simulink model "Grua_MC_R2_FFLimitado_06102026"  (R2025b)
settings: Solver=ode23t  StartTime=0.0  StopTime=628  MaxStep=T_s  RelTol=1e-4
InitFcn:
  | addpath(fileparts(get_param(bdroot,'FileName')),'-begin');
  | run(fullfile(fileparts(get_param(bdroot,'FileName')),'definir_buses_variadores.m'));
  | run(fullfile(fileparts(get_param(bdroot,'FileName')),'parametros_ganancias_cascada_29072026.m'));
  | run(fullfile(fileparts(get_param(bdroot,'FileName')),'configurar_modelo_final_hmi.m'));
  | run(fullfile(fileparts(get_param(bdroot,'FileName')),'configurar_parametros_variadores.m'));
  | Pvis.Ts_viz=.04;Pvis.enable=true;Pvis.keepFigureOnTerminate=true;Pvis.hmi.fastDiagnostic=false;
undefined symbols (not defined in the file or in its folder): b_cx, b_cy, b_hb, b_hEb, b_heq, b_t, b_tb, b_teq, b_tw, b_wu, g, H_c, HMI, i_h, i_t, J_heq, J_teq, K_cy, K_tw, k_wu, L_h0, l_hi, M_c_profile, M_s, M_t, MC_FF, nLevels0, omega_hmRATED, r_hd, r_td, slotBlock, T_hbMax, T_hEbMax, T_hmMax, T_s, T_s1, T_tbMax, T_tmMax, tau_hm, tau_tm, traj_duration, traj_x_start, traj_x_target, v_hmaxLoaded, v_hmaxUnloaded, x_tmax, x_tmin, Y_c0, Y_t0, Zbase
libraries: simulink x1, aerolibanimutils x1
(part 2 of 5)

== system Grua_MC_R2_FFLimitado_06102026/Actualizar_Yc ==
  tipo_evento : Inport
  slot_evento : Inport  Port=2
  Trigger : TriggerPort  VariantControl=(inherit)  PortDimensions=1
  Constant : Constant  Value=Zbase
  Constant1 : Constant  Value=slotBlock
  Constant2 : Constant  Value=H_c
  Unit Delay : UnitDelay  InitialCondition=nLevels0  SampleTime=-1  HasFrameUpgradeWarning=on
  update_perfil_std : MATLAB Function  TreatAsAtomicUnit=on
  Y_c : Outport  InitialOutput=Y_c0
  wires:
  update_perfil_std/2(Y_c) -> Y_c/1
  slot_evento/1 -> update_perfil_std/3(slot_evento)
  update_perfil_std/1(nLevels_new) -> Unit Delay/1
  tipo_evento/1 -> update_perfil_std/2(tipo_evento)
  Unit Delay/1 -> update_perfil_std/1(nLevels)
  Constant/1 -> update_perfil_std/4(Zbase)
  Constant1/1 -> update_perfil_std/5(slotBlock)
  Constant2/1 -> update_perfil_std/6(h_std)

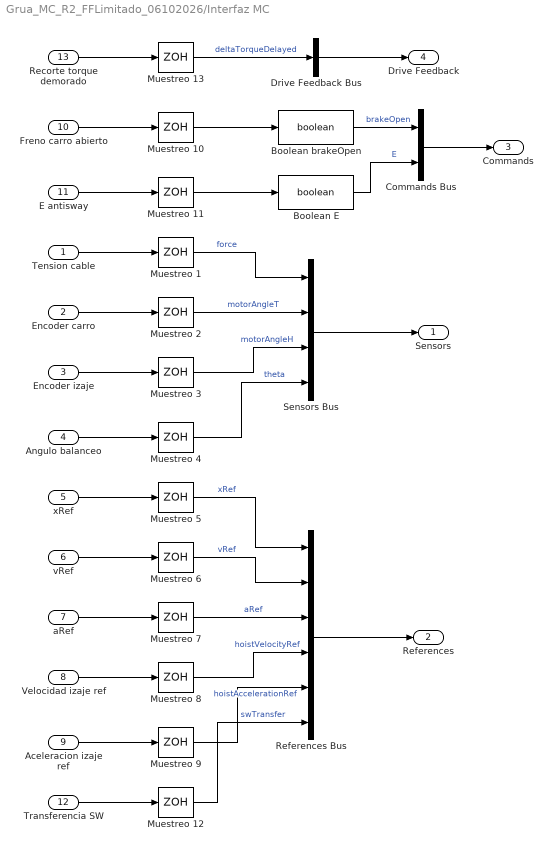
== system Grua_MC_R2_FFLimitado_06102026/Interfaz MC ==
  Tension cable : Inport
  Encoder carro : Inport  Port=2
  Encoder izaje : Inport  Port=3
  Angulo balanceo : Inport  Port=4
  xRef : Inport  Port=5
  vRef : Inport  Port=6
  aRef : Inport  Port=7
  Velocidad izaje ref : Inport  Port=8
  Aceleracion izaje ref : Inport  Port=9
  Freno carro abierto : Inport  Port=10
  E antisway : Inport  Port=11
  Transferencia SW : Inport  Port=12
  Recorte torque demorado : Inport  Port=13
  Boolean E : DataTypeConversion  OutDataTypeStr=boolean  SaturateOnIntegerOverflow=off  RndMeth=Floor
  Boolean brakeOpen : DataTypeConversion  OutDataTypeStr=boolean  SaturateOnIntegerOverflow=off  RndMeth=Floor
  Commands Bus : BusCreator  Inputs=2  OutDataTypeStr=Bus: MCFF_Commands  NonVirtualBus=on
  Drive Feedback Bus : BusCreator  Inputs=1  OutDataTypeStr=Bus: MCFF_DriveFeedback  NonVirtualBus=on
  Muestreo {1..13} (13 alike) : ZeroOrderHold  SampleTime=T_s
  References Bus : BusCreator  Inputs=6  OutDataTypeStr=Bus: MCFF_References  NonVirtualBus=on
  Sensors Bus : BusCreator  Inputs=4  OutDataTypeStr=Bus: MCFF_Sensors  NonVirtualBus=on
  Sensors : Outport
  References : Outport  Port=2
  Commands : Outport  Port=3
  Drive Feedback : Outport  Port=4
  wires:
  Drive Feedback Bus/1 -> Drive Feedback/1
  Muestreo 4/1 -> Sensors Bus/4  "theta"
  E antisway/1 -> Muestreo 11/1
  Recorte torque demorado/1 -> Muestreo 13/1
  Encoder carro/1 -> Muestreo 2/1
  Tension cable/1 -> Muestreo 1/1
  Muestreo 3/1 -> Sensors Bus/3  "motorAngleH"
  Freno carro abierto/1 -> Muestreo 10/1
  xRef/1 -> Muestreo 5/1
  Angulo balanceo/1 -> Muestreo 4/1
  Muestreo 11/1 -> Boolean E/1
  Encoder izaje/1 -> Muestreo 3/1
  Commands Bus/1 -> Commands/1
  vRef/1 -> Muestreo 6/1
  Boolean E/1 -> Commands Bus/2  "E"
  aRef/1 -> Muestreo 7/1
  Velocidad izaje ref/1 -> Muestreo 8/1
  Aceleracion izaje ref/1 -> Muestreo 9/1
  Transferencia SW/1 -> Muestreo 12/1
  Muestreo 13/1 -> Drive Feedback Bus/1  "deltaTorqueDelayed"
  Muestreo 10/1 -> Boolean brakeOpen/1
  Muestreo 1/1 -> Sensors Bus/1  "force"
  Muestreo 2/1 -> Sensors Bus/2  "motorAngleT"
  Muestreo 5/1 -> References Bus/1  "xRef"
  Muestreo 6/1 -> References Bus/2  "vRef"
  Muestreo 7/1 -> References Bus/3  "aRef"
  Muestreo 8/1 -> References Bus/4  "hoistVelocityRef"
  Muestreo 9/1 -> References Bus/5  "hoistAccelerationRef"
  Muestreo 12/1 -> References Bus/6  "swTransfer"
  Boolean brakeOpen/1 -> Commands Bus/1  "brakeOpen"
  Sensors Bus/1 -> Sensors/1
  References Bus/1 -> References/1

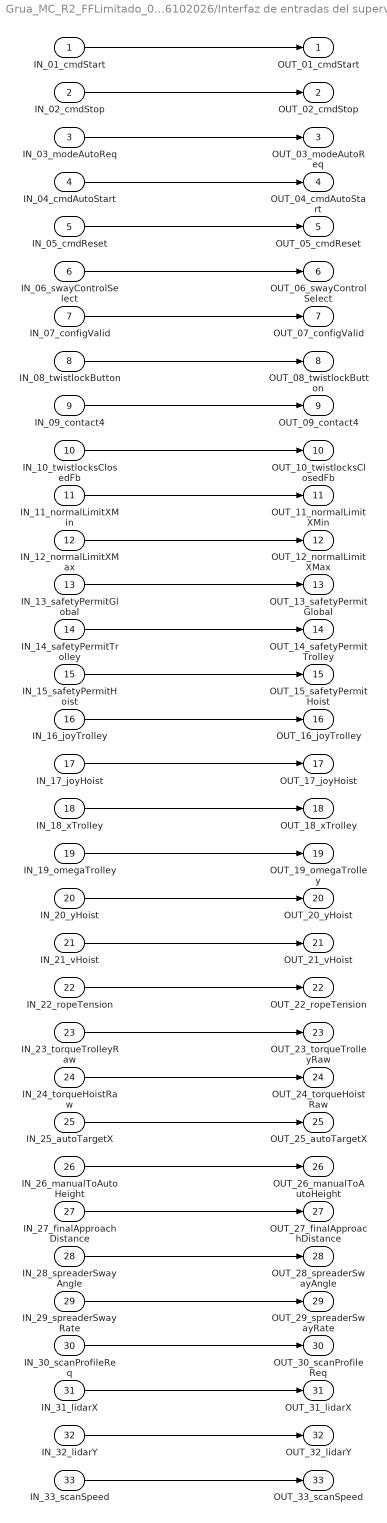
== system Grua_MC_R2_FFLimitado_06102026/Interfaz de entradas del supervisor ==
  IN_01_cmdStart : Inport
  IN_02_cmdStop : Inport  Port=2
  IN_03_modeAutoReq : Inport  Port=3
  IN_04_cmdAutoStart : Inport  Port=4
  IN_05_cmdReset : Inport  Port=5
  IN_06_swayControlSelect : Inport  Port=6
  IN_07_configValid : Inport  Port=7
  IN_08_twistlockButton : Inport  Port=8
  IN_09_contact4 : Inport  Port=9
  IN_10_twistlocksClosedFb : Inport  Port=10
  IN_11_normalLimitXMin : Inport  Port=11
  IN_12_normalLimitXMax : Inport  Port=12
  IN_13_safetyPermitGlobal : Inport  Port=13
  IN_14_safetyPermitTrolley : Inport  Port=14
  IN_15_safetyPermitHoist : Inport  Port=15
  IN_16_joyTrolley : Inport  Port=16
  IN_17_joyHoist : Inport  Port=17
  IN_18_xTrolley : Inport  Port=18
  IN_19_omegaTrolley : Inport  Port=19
  IN_20_yHoist : Inport  Port=20
  IN_21_vHoist : Inport  Port=21
  IN_22_ropeTension : Inport  Port=22
  IN_23_torqueTrolleyRaw : Inport  Port=23
  IN_24_torqueHoistRaw : Inport  Port=24
  IN_25_autoTargetX : Inport  Port=25
  IN_26_manualToAutoHeight : Inport  Port=26
  IN_27_finalApproachDistance : Inport  Port=27
  IN_28_spreaderSwayAngle : Inport  Port=28
  IN_29_spreaderSwayRate : Inport  Port=29
  IN_30_scanProfileReq : Inport  Port=30
  IN_31_lidarX : Inport  Port=31
  IN_32_lidarY : Inport  Port=32
  IN_33_scanSpeed : Inport  Port=33
  OUT_01_cmdStart : Outport
  OUT_02_cmdStop : Outport  Port=2
  OUT_03_modeAutoReq : Outport  Port=3
  OUT_04_cmdAutoStart : Outport  Port=4
  OUT_05_cmdReset : Outport  Port=5
  OUT_06_swayControlSelect : Outport  Port=6
  OUT_07_configValid : Outport  Port=7
  OUT_08_twistlockButton : Outport  Port=8
  OUT_09_contact4 : Outport  Port=9
  OUT_10_twistlocksClosedFb : Outport  Port=10
  OUT_11_normalLimitXMin : Outport  Port=11
  OUT_12_normalLimitXMax : Outport  Port=12
  OUT_13_safetyPermitGlobal : Outport  Port=13
  OUT_14_safetyPermitTrolley : Outport  Port=14
  OUT_15_safetyPermitHoist : Outport  Port=15
  OUT_16_joyTrolley : Outport  Port=16
  OUT_17_joyHoist : Outport  Port=17
  OUT_18_xTrolley : Outport  Port=18
  OUT_19_omegaTrolley : Outport  Port=19
  OUT_20_yHoist : Outport  Port=20
  OUT_21_vHoist : Outport  Port=21
  OUT_22_ropeTension : Outport  Port=22
  OUT_23_torqueTrolleyRaw : Outport  Port=23
  OUT_24_torqueHoistRaw : Outport  Port=24
  OUT_25_autoTargetX : Outport  Port=25
  OUT_26_manualToAutoHeight : Outport  Port=26
  OUT_27_finalApproachDistance : Outport  Port=27
  OUT_28_spreaderSwayAngle : Outport  Port=28
  OUT_29_spreaderSwayRate : Outport  Port=29
  OUT_30_scanProfileReq : Outport  Port=30
  OUT_31_lidarX : Outport  Port=31
  OUT_32_lidarY : Outport  Port=32
  OUT_33_scanSpeed : Outport  Port=33
  wires:
  IN_01_cmdStart/1 -> OUT_01_cmdStart/1
  IN_02_cmdStop/1 -> OUT_02_cmdStop/1
  IN_03_modeAutoReq/1 -> OUT_03_modeAutoReq/1
  IN_04_cmdAutoStart/1 -> OUT_04_cmdAutoStart/1
  IN_05_cmdReset/1 -> OUT_05_cmdReset/1
  IN_06_swayControlSelect/1 -> OUT_06_swayControlSelect/1
  IN_07_configValid/1 -> OUT_07_configValid/1
  IN_08_twistlockButton/1 -> OUT_08_twistlockButton/1
  IN_09_contact4/1 -> OUT_09_contact4/1
  IN_10_twistlocksClosedFb/1 -> OUT_10_twistlocksClosedFb/1
  IN_11_normalLimitXMin/1 -> OUT_11_normalLimitXMin/1
  IN_12_normalLimitXMax/1 -> OUT_12_normalLimitXMax/1
  IN_13_safetyPermitGlobal/1 -> OUT_13_safetyPermitGlobal/1
  IN_14_safetyPermitTrolley/1 -> OUT_14_safetyPermitTrolley/1
  IN_15_safetyPermitHoist/1 -> OUT_15_safetyPermitHoist/1
  IN_16_joyTrolley/1 -> OUT_16_joyTrolley/1
  IN_17_joyHoist/1 -> OUT_17_joyHoist/1
  IN_18_xTrolley/1 -> OUT_18_xTrolley/1
  IN_19_omegaTrolley/1 -> OUT_19_omegaTrolley/1
  IN_20_yHoist/1 -> OUT_20_yHoist/1
  IN_21_vHoist/1 -> OUT_21_vHoist/1
  IN_22_ropeTension/1 -> OUT_22_ropeTension/1
  IN_23_torqueTrolleyRaw/1 -> OUT_23_torqueTrolleyRaw/1
  IN_24_torqueHoistRaw/1 -> OUT_24_torqueHoistRaw/1
  IN_25_autoTargetX/1 -> OUT_25_autoTargetX/1
  IN_26_manualToAutoHeight/1 -> OUT_26_manualToAutoHeight/1
  IN_27_finalApproachDistance/1 -> OUT_27_finalApproachDistance/1
  IN_28_spreaderSwayAngle/1 -> OUT_28_spreaderSwayAngle/1
  IN_29_spreaderSwayRate/1 -> OUT_29_spreaderSwayRate/1
  IN_30_scanProfileReq/1 -> OUT_30_scanProfileReq/1
  IN_31_lidarX/1 -> OUT_31_lidarX/1
  IN_32_lidarY/1 -> OUT_32_lidarY/1
  IN_33_scanSpeed/1 -> OUT_33_scanSpeed/1

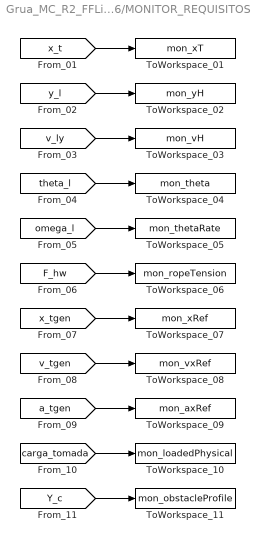
== system Grua_MC_R2_FFLimitado_06102026/MONITOR_REQUISITOS ==
  ToWorkspace_01 : ToWorkspace  VariableName=mon_xT  SaveFormat=Timeseries  SampleTime=-1
      settings: Decimation=10
  ToWorkspace_02 : ToWorkspace  VariableName=mon_yH  SaveFormat=Timeseries  SampleTime=-1
      settings: Decimation=10
  ToWorkspace_03 : ToWorkspace  VariableName=mon_vH  SaveFormat=Timeseries  SampleTime=-1
      settings: Decimation=10
  ToWorkspace_04 : ToWorkspace  VariableName=mon_theta  SaveFormat=Timeseries  SampleTime=-1
      settings: Decimation=10
  ToWorkspace_05 : ToWorkspace  VariableName=mon_thetaRate  SaveFormat=Timeseries  SampleTime=-1
      settings: Decimation=10
  ToWorkspace_06 : ToWorkspace  VariableName=mon_ropeTension  SaveFormat=Timeseries  SampleTime=-1
      settings: Decimation=10
  ToWorkspace_07 : ToWorkspace  VariableName=mon_xRef  SaveFormat=Timeseries  SampleTime=-1
      settings: Decimation=10
  ToWorkspace_08 : ToWorkspace  VariableName=mon_vxRef  SaveFormat=Timeseries  SampleTime=-1
      settings: Decimation=10
  ToWorkspace_09 : ToWorkspace  VariableName=mon_axRef  SaveFormat=Timeseries  SampleTime=-1
      settings: Decimation=10
  ToWorkspace_10 : ToWorkspace  VariableName=mon_loadedPhysical  SaveFormat=Timeseries  SampleTime=-1
      settings: Decimation=10
  ToWorkspace_11 : ToWorkspace  VariableName=mon_obstacleProfile  SaveFormat=Timeseries  SampleTime=-1
      settings: Decimation=10
  wires:
  [x_t] -> ToWorkspace_01/1
  [y_l] -> ToWorkspace_02/1
  [v_ly] -> ToWorkspace_03/1
  [theta_l] -> ToWorkspace_04/1
  [omega_l] -> ToWorkspace_05/1
  [F_hw] -> ToWorkspace_06/1
  [x_tgen] -> ToWorkspace_07/1
  [v_tgen] -> ToWorkspace_08/1
  [a_tgen] -> ToWorkspace_09/1
  [carga_tomada] -> ToWorkspace_10/1
  [Y_c] -> ToWorkspace_11/1

== system Grua_MC_R2_FFLimitado_06102026/Motion Controller ==
  Sensors : Inport  OutDataTypeStr=Bus: MCFF_Sensors
  References : Inport  Port=2  OutDataTypeStr=Bus: MCFF_References
  Commands : Inport  Port=3  OutDataTypeStr=Bus: MCFF_Commands
  Drive Feedback : Inport  Port=4  OutDataTypeStr=Bus: MCFF_DriveFeedback
  Diagnosticos : Subsystem
  Estimadores : MATLAB Function  TreatAsAtomicUnit=on
  MC Carro : MATLAB Function  TreatAsAtomicUnit=on
  MC Izaje : MATLAB Function  TreatAsAtomicUnit=on
  Parameters : Constant  Value=MC_FF  OutDataTypeStr=Bus: MCFF_Parameters  SampleTime=T_s
  T_hm* : Outport
  T_tmcontrolador : Outport  Port=2
  SW aplicada comun : Outport  Port=3
  Estados carro : Outport  Port=4
  Estados izaje : Outport  Port=5
  Diagnosticos carro : Outport  Port=6
  Diagnosticos izaje : Outport  Port=7
  wires:
  MC Carro/1(torque) -> T_tmcontrolador/1
  Sensors/1 -> MC Carro/1(s), MC Izaje/1(s), Estimadores/1(s)
  Parameters/1 -> MC Carro/7(p), MC Izaje/4(p), Estimadores/2(p)
  MC Carro/2(sw) -> SW aplicada comun/1
  Commands/1 -> MC Carro/3(c)
  Drive Feedback/1 -> MC Carro/4(drive)
  Estimadores/1(cart) -> MC Carro/5(est), Estados carro/1
  References/1 -> MC Carro/2(r), MC Izaje/2(r)
  Estimadores/2(hoist) -> MC Izaje/3(est), MC Carro/6(hoist), Estados izaje/1
  MC Carro/3(d) -> Diagnosticos/1(In1), Diagnosticos carro/1
  MC Izaje/1(torque) -> T_hm*/1
  MC Izaje/2(d) -> Diagnosticos izaje/1, Diagnosticos/2(In2)

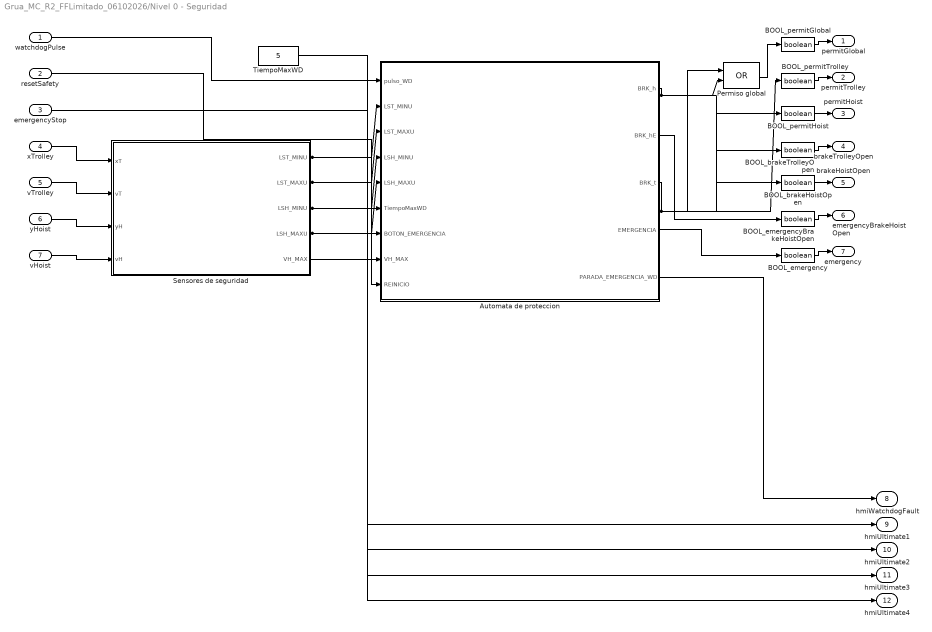
== system Grua_MC_R2_FFLimitado_06102026/Nivel 0 - Seguridad ==
  watchdogPulse : Inport
  resetSafety : Inport  Port=2
  emergencyStop : Inport  Port=3
  xTrolley : Inport  Port=4
  vTrolley : Inport  Port=5
  yHoist : Inport  Port=6
  vHoist : Inport  Port=7
  Automata de proteccion : Stateflow chart  TreatAsAtomicUnit=on
      settings: PortSchema="{\"entries\":[{\"content\":{\"sides\":[{\"content\":{\"connectorIds\":[\"In1\",\"In3\",\"In4\",\"In5\",\"In6\",\"In7\",\"In8\",\"In9\",\"In2\"]},\"type\":\"ConnectorPlacement.EquallySpacedRectSide\",\"uuid\":\"cd0792a4-97ef-4c80-9019-d76753964359\"},{\"content\":{\"connectorIds\":[\"Out1\",\"Out2\",\"Out3\",\"Out4\",\"Out5\"],\"side\":\"RIGHT\"},\"type\":\"ConnectorPlacement.EquallySpacedRectSide\",\"uuid\":\"2986dd5d-2111-4155-8673-f52c044c46ad\"},{\"content\":{\"side\":\"TOP\"},\"type\":\"ConnectorPlacement.EquallySpacedRectSide\",\"uuid\":\"d52e82c5-c118-49d3-899a-ea936e299c34\"}]},\"type\":\"ConnectorPlacement.EquallySpacedConnector\",\"uuid\":\"580a1a82-6a30-4652-9187-78ca47e5d1d9\"}],\"packageUris\":[\"http://schema.mathworks.com/mf0/Connector/R2020b\"],\"version\":\"1.0\"}"
  BOOL_brakeHoistOpen : DataTypeConversion  OutDataTypeStr=boolean  SaturateOnIntegerOverflow=off  RndMeth=Floor
  BOOL_brakeTrolleyOpen : DataTypeConversion  OutDataTypeStr=boolean  SaturateOnIntegerOverflow=off  RndMeth=Floor
  BOOL_emergency : DataTypeConversion  OutDataTypeStr=boolean  SaturateOnIntegerOverflow=off  RndMeth=Floor
  BOOL_emergencyBrakeHoistOpen : DataTypeConversion  OutDataTypeStr=boolean  SaturateOnIntegerOverflow=off  RndMeth=Floor
  BOOL_permitGlobal : DataTypeConversion  OutDataTypeStr=boolean  SaturateOnIntegerOverflow=off  RndMeth=Floor
  BOOL_permitHoist : DataTypeConversion  OutDataTypeStr=boolean  SaturateOnIntegerOverflow=off  RndMeth=Floor
  BOOL_permitTrolley : DataTypeConversion  OutDataTypeStr=boolean  SaturateOnIntegerOverflow=off  RndMeth=Floor
  Permiso global : Logic  Operator=OR  AllPortsSameDT=off  OutDataTypeStr=boolean
  Sensores de seguridad : MATLAB Function  TreatAsAtomicUnit=on
  TiempoMaxWD : Constant  Value=5  OutDataTypeStr=double
  permitGlobal : Outport
  permitTrolley : Outport  Port=2
  permitHoist : Outport  Port=3
  brakeTrolleyOpen : Outport  Port=4
  brakeHoistOpen : Outport  Port=5
  emergencyBrakeHoistOpen : Outport  Port=6
  emergency : Outport  Port=7
  hmiWatchdogFault : Outport  Port=8
  hmiUltimate1 : Outport  Port=9
  hmiUltimate2 : Outport  Port=10
  hmiUltimate3 : Outport  Port=11
  hmiUltimate4 : Outport  Port=12
  wires:
  xTrolley/1 -> Sensores de seguridad/1(xT)
  vTrolley/1 -> Sensores de seguridad/2(vT)
  yHoist/1 -> Sensores de seguridad/3(yH)
  vHoist/1 -> Sensores de seguridad/4(vH)
  watchdogPulse/1 -> Automata de proteccion/1(pulso_WD)
  resetSafety/1 -> Automata de proteccion/2(REINICIO)
  Sensores de seguridad/1(LST_MINU) -> Automata de proteccion/3(LST_MINU), hmiUltimate1/1
  Sensores de seguridad/2(LST_MAXU) -> Automata de proteccion/4(LST_MAXU), hmiUltimate2/1
  Sensores de seguridad/3(LSH_MINU) -> Automata de proteccion/5(LSH_MINU), hmiUltimate3/1
  Sensores de seguridad/4(LSH_MAXU) -> Automata de proteccion/6(LSH_MAXU), hmiUltimate4/1
  TiempoMaxWD/1 -> Automata de proteccion/7(TiempoMaxWD)
  emergencyStop/1 -> Automata de proteccion/8(BOTON_EMERGENCIA)
  Sensores de seguridad/5(VH_MAX) -> Automata de proteccion/9(VH_MAX)
  Automata de proteccion/3(BRK_t) -> Permiso global/1, BOOL_permitTrolley/1, BOOL_brakeTrolleyOpen/1
  Automata de proteccion/1(BRK_h) -> Permiso global/2, BOOL_permitHoist/1, BOOL_brakeHoistOpen/1
  Permiso global/1 -> BOOL_permitGlobal/1
  BOOL_permitGlobal/1 -> permitGlobal/1
  BOOL_permitTrolley/1 -> permitTrolley/1
  BOOL_permitHoist/1 -> permitHoist/1
  BOOL_brakeTrolleyOpen/1 -> brakeTrolleyOpen/1
  BOOL_brakeHoistOpen/1 -> brakeHoistOpen/1
  Automata de proteccion/2(BRK_hE) -> BOOL_emergencyBrakeHoistOpen/1
  BOOL_emergencyBrakeHoistOpen/1 -> emergencyBrakeHoistOpen/1
  Automata de proteccion/4(EMERGENCIA) -> BOOL_emergency/1
  BOOL_emergency/1 -> emergency/1
  Automata de proteccion/5(PARADA_EMERGENCIA_WD) -> hmiWatchdogFault/1

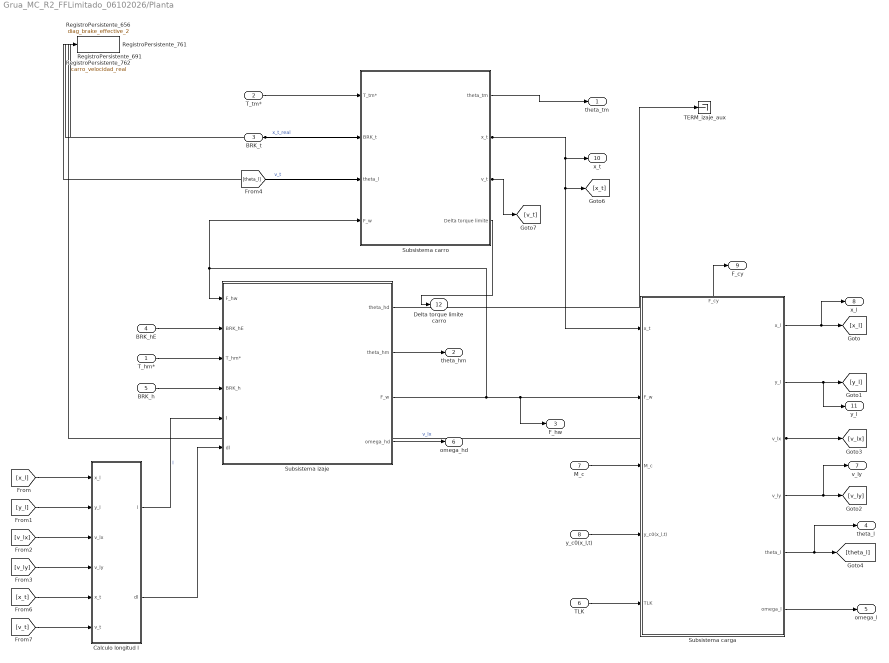
== system Grua_MC_R2_FFLimitado_06102026/Planta ==
  T_hm* : Inport
  T_tm* : Inport  Port=2
  BRK_t : Inport  Port=3
  BRK_hE : Inport  Port=4
  BRK_h : Inport  Port=5
  TLK : Inport  Port=6
  M_c : Inport  Port=7
  y_c0(x_l,t) : Inport  Port=8
  Calculo longitud l : Subsystem
  RegistroPersistente_656 : ToWorkspace  VariableName=diag_brake_effective_2  SaveFormat=Timeseries  SampleTime=-1
      settings: Decimation=10
  RegistroPersistente_691 : ToWorkspace  VariableName=v_lx  SaveFormat=Timeseries  SampleTime=-1
      settings: Decimation=10
  RegistroPersistente_761 : ToWorkspace  VariableName=x_t_real  SaveFormat=Timeseries  SampleTime=-1
      settings: Decimation=10
  RegistroPersistente_762 : ToWorkspace  VariableName=carro_velocidad_real  SaveFormat=Timeseries  SampleTime=-1
      settings: Decimation=10
  Subsistema carga : Subsystem
      settings: PortSchema="{\"entries\":[{\"content\":{\"sides\":[{\"content\":{\"connectorIds\":[\"In1\",\"In2\",\"In3\",\"In4\",\"In5\"]},\"type\":\"ConnectorPlacement.EquallySpacedRectSide\",\"uuid\":\"47edabbd-243a-4b83-941f-e4392c1d00a7\"},{\"content\":{\"connectorIds\":[\"Out1\",\"Out2\",\"Out3\",\"Out4\",\"Out5\",\"Out6\"],\"side\":\"RIGHT\"},\"type\":\"ConnectorPlacement.EquallySpacedRectSide\",\"uuid\":\"f3c5bb4b-ba1f-46ef-b9da-f46dde7ba679\"},{\"content\":{\"connectorIds\":[\"Out7\"],\"side\":\"TOP\"},\"type\":\"ConnectorPlacement.EquallySpacedRectSide\",\"uuid\":\"99c64c8e-1061-494c-a8fc-4982bc564791\"}]},\"type\":\"ConnectorPlacement.EquallySpacedConnector\",\"uuid\":\"f8d59f7d-b4a0-41b3-9b68-cb1adbf574c0\"}],\"packageUris\":[\"http://schema.mathworks.com/mf0/Connector/R2020b\"],\"version\":\"1.0\"}"
  Subsistema carro : Subsystem
  Subsistema izaje : Subsystem
  TERM_izaje_aux : Terminator
  theta_tm : Outport
  theta_hm : Outport  Port=2
  F_hw : Outport  Port=3
  theta_l : Outport  Port=4
  omega_l : Outport  Port=5
  omega_hd : Outport  Port=6
  v_ly : Outport  Port=7
  x_l : Outport  Port=8
  F_cy : Outport  Port=9
  x_t : Outport  Port=10
  y_l : Outport  Port=11
  Delta torque limite carro : Outport  Port=12
  wires:
  y_c0(x_l,t)/1 -> Subsistema carga/4(y_c0(x_l,t))
  [x_t] -> Calculo longitud l/5(x_t)
  Subsistema izaje/3(F_w) -> Subsistema carro/4(F_w), Subsistema izaje/1(F_hw), F_hw/1, Subsistema carga/2(F_w)
  Subsistema carro/2(x_t) -> x_t/1, Subsistema carga/1(x_t), [x_t], RegistroPersistente_761/1  "x_t_real"
  [y_l] -> Calculo longitud l/2(y_l)
  BRK_hE/1 -> Subsistema izaje/2(BRK_hE)
  T_hm*/1 -> Subsistema izaje/3(T_hm*)
  T_tm*/1 -> Subsistema carro/1(T_tm*)
  Subsistema carga/3(v_lx) -> [v_lx], RegistroPersistente_691/1  "v_lx"
  [v_ly] -> Calculo longitud l/4(v_ly)
  Subsistema carga/2(y_l) -> [y_l], y_l/1
  Subsistema carga/4(v_ly) -> v_ly/1, [v_ly]
  Subsistema carga/1(x_l) -> x_l/1, [x_l]
  Subsistema carga/6(omega_l) -> omega_l/1
  [theta_l] -> Subsistema carro/3(theta_l)
  Calculo longitud l/2(dl) -> Subsistema izaje/6(dl)
  [v_lx] -> Calculo longitud l/3(v_lx)
  BRK_t/1 -> Subsistema carro/2(BRK_t), RegistroPersistente_656/1
  M_c/1 -> Subsistema carga/3(M_c)
  [x_l] -> Calculo longitud l/1(x_l)
  Subsistema carro/3(v_t) -> [v_t], RegistroPersistente_762/1  "v_t"
  Calculo longitud l/1(l) -> Subsistema izaje/5(l)  "l"
  [v_t] -> Calculo longitud l/6(v_t)
  BRK_h/1 -> Subsistema izaje/4(BRK_h)
  Subsistema izaje/4(omega_hd) -> omega_hd/1
  Subsistema carro/1(theta_tm) -> theta_tm/1
  Subsistema izaje/2(theta_hm) -> theta_hm/1
  Subsistema carga/5(theta_l) -> theta_l/1, [theta_l]
  Subsistema carga/7(F_cy) -> F_cy/1
  TLK/1 -> Subsistema carga/5(TLK)
  Subsistema izaje/1(theta_hd) -> TERM_izaje_aux/1
  Subsistema carro/4(Delta torque limite) -> Delta torque limite carro/1

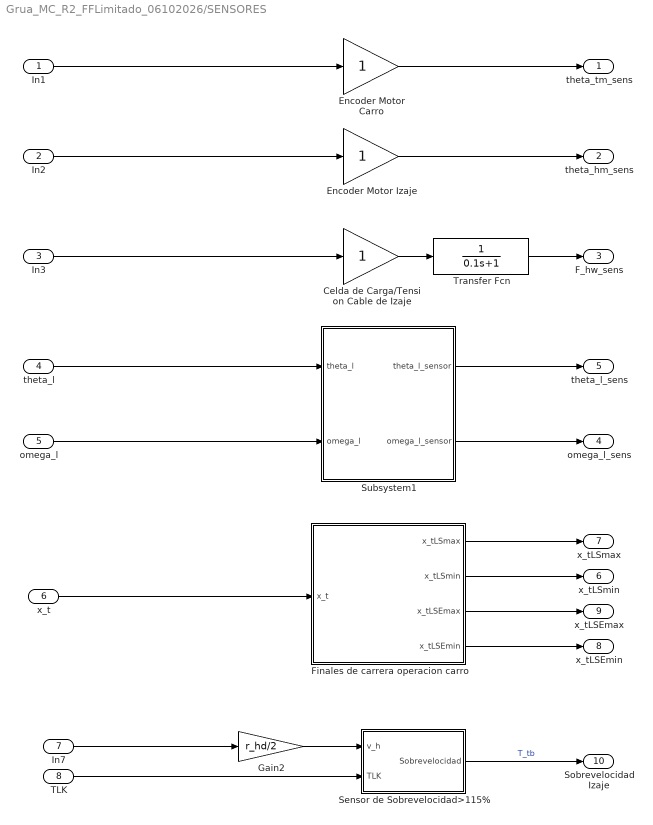
== system Grua_MC_R2_FFLimitado_06102026/SENSORES ==
  In1 : Inport
  In2 : Inport  Port=2
  In3 : Inport  Port=3
  theta_l : Inport  Port=4
  omega_l : Inport  Port=5
  x_t : Inport  Port=6
  In7 : Inport  Port=7
  TLK : Inport  Port=8
  Celda de Carga/Tension Cable de Izaje : Gain
  Encoder Motor Carro : Gain
  Encoder Motor Izaje : Gain
  Finales de carrera operacion carro : Subsystem
  Gain2 : Gain  Gain=r_hd/2
  Sensor de Sobrevelocidad>115% : Subsystem
  Subsystem1 : Subsystem
  Transfer Fcn : TransferFcn  Denominator=[0.1 1]
  theta_tm_sens : Outport
  theta_hm_sens : Outport  Port=2
  F_hw_sens : Outport  Port=3
  omega_l_sens : Outport  Port=4
  theta_l_sens : Outport  Port=5
  x_tLSmin : Outport  Port=6
  x_tLSmax : Outport  Port=7
  x_tLSEmin : Outport  Port=8
  x_tLSEmax : Outport  Port=9
  Sobrevelocidad Izaje : Outport  Port=10
  wires:
  In1/1 -> Encoder Motor Carro/1
  Finales de carrera operacion carro/2(x_tLSmin) -> x_tLSmin/1
  Finales de carrera operacion carro/4(x_tLSEmin) -> x_tLSEmin/1
  Finales de carrera operacion carro/3(x_tLSEmax) -> x_tLSEmax/1
  Celda de Carga/Tension Cable de Izaje/1 -> Transfer Fcn/1
  Subsystem1/2(omega_l_sensor) -> omega_l_sens/1
  Encoder Motor Carro/1 -> theta_tm_sens/1
  Subsystem1/1(theta_l_sensor) -> theta_l_sens/1
  Sensor de Sobrevelocidad>115%/1(Sobrevelocidad) -> Sobrevelocidad Izaje/1  "T_tb"
  Gain2/1 -> Sensor de Sobrevelocidad>115%/1(v_h)
  x_t/1 -> Finales de carrera operacion carro/1(x_t)
  Encoder Motor Izaje/1 -> theta_hm_sens/1
  Finales de carrera operacion carro/1(x_tLSmax) -> x_tLSmax/1
  TLK/1 -> Sensor de Sobrevelocidad>115%/2(TLK)
  theta_l/1 -> Subsystem1/1(theta_l)
  In3/1 -> Celda de Carga/Tension Cable de Izaje/1
  omega_l/1 -> Subsystem1/2(omega_l)
  In2/1 -> Encoder Motor Izaje/1
  In7/1 -> Gain2/1
  Transfer Fcn/1 -> F_hw_sens/1

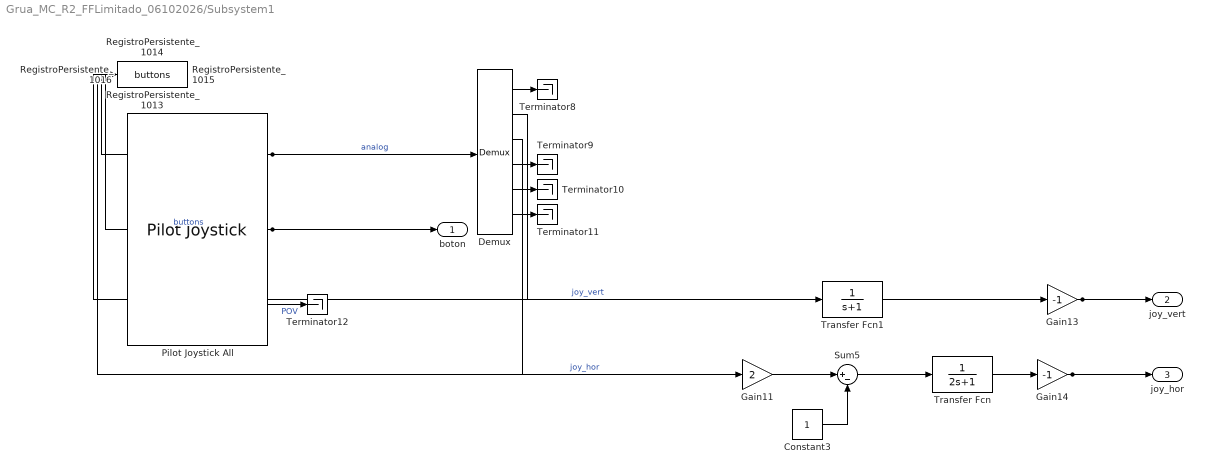
== system Grua_MC_R2_FFLimitado_06102026/Subsystem1 ==
  Constant3 : Constant
  Demux : Demux  Outputs=6
  Gain11 : Gain  Gain=2
  Gain13 : Gain  Gain=-1
  Gain14 : Gain  Gain=-1
  Pilot Joystick All : aerolibanimutils/Pilot Joystick  JoystickID=None  OutputConfiguration=AllOutputs  SampleTime=1/3000
      settings: LibrarySourceBlock=aerolibanimutils/Pilot Joystick All
  RegistroPersistente_1013 : ToWorkspace  VariableName=joy_vert  SaveFormat=Timeseries  SampleTime=-1
      settings: Decimation=10
  RegistroPersistente_1014 : ToWorkspace  VariableName=joy_hor  SaveFormat=Timeseries  SampleTime=-1
      settings: Decimation=10
  RegistroPersistente_1015 : ToWorkspace  VariableName=analog  SaveFormat=Timeseries  SampleTime=-1
      settings: Decimation=10
  RegistroPersistente_1016 : ToWorkspace  VariableName=buttons  SaveFormat=Timeseries  SampleTime=-1
      settings: Decimation=10
  Sum5 : Sum  Inputs=|+-
  Terminator{8..12} (5 alike) : Terminator
  Transfer Fcn : TransferFcn  Denominator=[2 1]
  Transfer Fcn1 : TransferFcn  Denominator=[1 1]
  boton : Outport
  joy_vert : Outport  Port=2
  joy_hor : Outport  Port=3
  wires:
  Demux/5 -> Terminator10/1
  Pilot Joystick All/2 -> boton/1, RegistroPersistente_1016/1  "buttons"
  Demux/2 -> Transfer Fcn1/1
  Constant3/1 -> Sum5/2
  Pilot Joystick All/3 -> Terminator12/1  "POV"
  Transfer Fcn/1 -> Gain14/1
  Demux/1 -> Terminator8/1
  Sum5/1 -> Transfer Fcn/1
  Gain11/1 -> Sum5/1
  Demux/3 -> Gain11/1
  Transfer Fcn1/1 -> Gain13/1
  Pilot Joystick All/1 -> Demux/1, RegistroPersistente_1015/1  "analog"
  Demux/4 -> Terminator9/1
  Demux/6 -> Terminator11/1
  Gain14/1 -> joy_hor/1, RegistroPersistente_1014/1  "joy_hor"
  Gain13/1 -> joy_vert/1, RegistroPersistente_1013/1  "joy_vert"

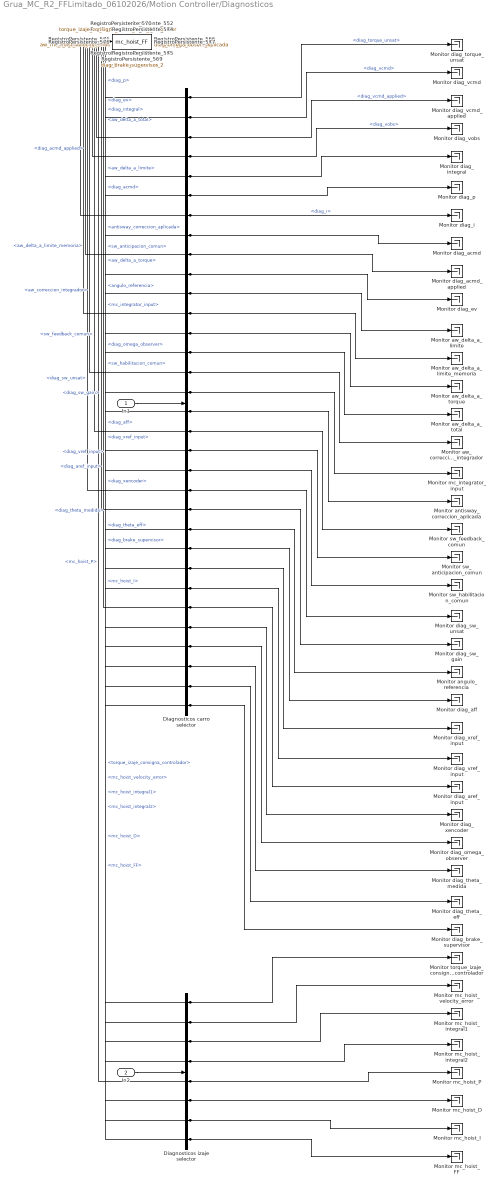
== system Grua_MC_R2_FFLimitado_06102026/Motion Controller/Diagnosticos ==
  In1 : Inport
  In2 : Inport  Port=2
  Diagnosticos carro selector : BusSelector  OutputSignals=diag_torque_unsat,diag_vcmd,diag_vcmd_applied,diag_vobs,diag_integral,diag_p,diag_i,diag_acmd,diag_acmd_applied,diag_ev,aw_delta_a_limite,aw_delta_a_limite_memoria,aw_delta_a_torque,aw_delta_a_total,aw_correccion_integrador,mc_integrator_input,antisway_correccion_aplicada,sw_feedback_comun,sw_anticipacion_comun,sw_habilitacion_comun,diag_sw_unsat,diag_sw_gain,angulo_referencia,diag_aff,diag_xref_input,diag_vref_input,diag_aref_input,diag_xencoder,diag_omega_observer,diag_theta_medida,diag_theta_eff,diag_brake_supervisor
  Diagnosticos izaje selector : BusSelector  OutputSignals=torque_izaje_consigna_controlador,mc_hoist_velocity_error,mc_hoist_integral1,mc_hoist_integral2,mc_hoist_P,mc_hoist_D,mc_hoist_I,mc_hoist_FF
  Monitor angulo_referencia : Terminator
  Monitor antisway_correccion_aplicada : Terminator
  Monitor aw_correccion_integrador : Terminator
  Monitor aw_delta_a_limite : Terminator
  Monitor aw_delta_a_limite_memoria : Terminator
  Monitor aw_delta_a_torque : Terminator
  Monitor aw_delta_a_total : Terminator
  Monitor diag_acmd : Terminator
  Monitor diag_acmd_applied : Terminator
  Monitor diag_aff : Terminator
  Monitor diag_aref_input : Terminator
  Monitor diag_brake_supervisor : Terminator
  Monitor diag_ev : Terminator
  Monitor diag_i : Terminator
  Monitor diag_integral : Terminator
  Monitor diag_omega_observer : Terminator
  Monitor diag_p : Terminator
  Monitor diag_sw_gain : Terminator
  Monitor diag_sw_unsat : Terminator
  Monitor diag_theta_eff : Terminator
  Monitor diag_theta_medida : Terminator
  Monitor diag_torque_unsat : Terminator
  Monitor diag_vcmd : Terminator
  Monitor diag_vcmd_applied : Terminator
  Monitor diag_vobs : Terminator
  Monitor diag_vref_input : Terminator
  Monitor diag_xencoder : Terminator
  Monitor diag_xref_input : Terminator
  Monitor mc_hoist_D : Terminator
  Monitor mc_hoist_FF : Terminator
  Monitor mc_hoist_I : Terminator
  Monitor mc_hoist_P : Terminator
  Monitor mc_hoist_integral1 : Terminator
  Monitor mc_hoist_integral2 : Terminator
  Monitor mc_hoist_velocity_error : Terminator
  Monitor mc_integrator_input : Terminator
  Monitor sw_anticipacion_comun : Terminator
  Monitor sw_feedback_comun : Terminator
  Monitor sw_habilitacion_comun : Terminator
  Monitor torque_izaje_consigna_controlador : Terminator
  RegistroPersistente_538 : ToWorkspace  VariableName=diag_torque_unsat  SaveFormat=Timeseries  SampleTime=-1
      settings: Decimation=10
  RegistroPersistente_539 : ToWorkspace  VariableName=diag_vcmd  SaveFormat=Timeseries  SampleTime=-1
      settings: Decimation=10
  RegistroPersistente_540 : ToWorkspace  VariableName=diag_vcmd_applied  SaveFormat=Timeseries  SampleTime=-1
      settings: Decimation=10
  RegistroPersistente_541 : ToWorkspace  VariableName=diag_vobs  SaveFormat=Timeseries  SampleTime=-1
      settings: Decimation=10
  RegistroPersistente_542 : ToWorkspace  VariableName=diag_integral  SaveFormat=Timeseries  SampleTime=-1
      settings: Decimation=10
  RegistroPersistente_543 : ToWorkspace  VariableName=diag_p  SaveFormat=Timeseries  SampleTime=-1
      settings: Decimation=10
  RegistroPersistente_544 : ToWorkspace  VariableName=diag_i  SaveFormat=Timeseries  SampleTime=-1
      settings: Decimation=10
  RegistroPersistente_545 : ToWorkspace  VariableName=diag_acmd  SaveFormat=Timeseries  SampleTime=-1
      settings: Decimation=10
  RegistroPersistente_546 : ToWorkspace  VariableName=diag_acmd_applied  SaveFormat=Timeseries  SampleTime=-1
      settings: Decimation=10
  RegistroPersistente_547 : ToWorkspace  VariableName=diag_ev  SaveFormat=Timeseries  SampleTime=-1
      settings: Decimation=10
  RegistroPersistente_548 : ToWorkspace  VariableName=aw_delta_a_limite  SaveFormat=Timeseries  SampleTime=-1
      settings: Decimation=10
  RegistroPersistente_549 : ToWorkspace  VariableName=aw_delta_a_limite_memoria  SaveFormat=Timeseries  SampleTime=-1
      settings: Decimation=10
  RegistroPersistente_550 : ToWorkspace  VariableName=aw_delta_a_torque  SaveFormat=Timeseries  SampleTime=-1
      settings: Decimation=10
  RegistroPersistente_551 : ToWorkspace  VariableName=aw_delta_a_total  SaveFormat=Timeseries  SampleTime=-1
      settings: Decimation=10
  RegistroPersistente_552 : ToWorkspace  VariableName=aw_correccion_integrador  SaveFormat=Timeseries  SampleTime=-1
      settings: Decimation=10
  RegistroPersistente_553 : ToWorkspace  VariableName=mc_integrator_input  SaveFormat=Timeseries  SampleTime=-1
      settings: Decimation=10
  RegistroPersistente_554 : ToWorkspace  VariableName=antisway_correccion_aplicada  SaveFormat=Timeseries  SampleTime=-1
      settings: Decimation=10
  RegistroPersistente_555 : ToWorkspace  VariableName=sw_feedback_comun  SaveFormat=Timeseries  SampleTime=-1
      settings: Decimation=10
  RegistroPersistente_556 : ToWorkspace  VariableName=sw_anticipacion_comun  SaveFormat=Timeseries  SampleTime=-1
      settings: Decimation=10
  RegistroPersistente_557 : ToWorkspace  VariableName=sw_habilitacion_comun  SaveFormat=Timeseries  SampleTime=-1
      settings: Decimation=10
  RegistroPersistente_558 : ToWorkspace  VariableName=diag_sw_unsat  SaveFormat=Timeseries  SampleTime=-1
      settings: Decimation=10
  RegistroPersistente_559 : ToWorkspace  VariableName=diag_sw_gain  SaveFormat=Timeseries  SampleTime=-1
      settings: Decimation=10
  RegistroPersistente_560 : ToWorkspace  VariableName=angulo_referencia  SaveFormat=Timeseries  SampleTime=-1
      settings: Decimation=10
  RegistroPersistente_561 : ToWorkspace  VariableName=diag_aff  SaveFormat=Timeseries  SampleTime=-1
      settings: Decimation=10
  RegistroPersistente_562 : ToWorkspace  VariableName=diag_xref_input_2  SaveFormat=Timeseries  SampleTime=-1
      settings: Decimation=10
  RegistroPersistente_563 : ToWorkspace  VariableName=diag_vref_input_2  SaveFormat=Timeseries  SampleTime=-1
      settings: Decimation=10
  RegistroPersistente_564 : ToWorkspace  VariableName=diag_aref_input_2  SaveFormat=Timeseries  SampleTime=-1
      settings: Decimation=10
  RegistroPersistente_565 : ToWorkspace  VariableName=diag_xencoder  SaveFormat=Timeseries  SampleTime=-1
      settings: Decimation=10
  RegistroPersistente_566 : ToWorkspace  VariableName=diag_omega_observer  SaveFormat=Timeseries  SampleTime=-1
      settings: Decimation=10
  RegistroPersistente_567 : ToWorkspace  VariableName=diag_theta_medida  SaveFormat=Timeseries  SampleTime=-1
      settings: Decimation=10
  RegistroPersistente_568 : ToWorkspace  VariableName=diag_theta_eff  SaveFormat=Timeseries  SampleTime=-1
      settings: Decimation=10
  RegistroPersistente_569 : ToWorkspace  VariableName=diag_brake_supervisor_2  SaveFormat=Timeseries  SampleTime=-1
      settings: Decimation=10
  RegistroPersistente_570 : ToWorkspace  VariableName=torque_izaje_consigna_controlador_2  SaveFormat=Timeseries  SampleTime=-1
      settings: Decimation=10
  RegistroPersistente_571 : ToWorkspace  VariableName=mc_hoist_velocity_error  SaveFormat=Timeseries  SampleTime=-1
      settings: Decimation=10
  RegistroPersistente_572 : ToWorkspace  VariableName=mc_hoist_integral1  SaveFormat=Timeseries  SampleTime=-1
      settings: Decimation=10
  RegistroPersistente_573 : ToWorkspace  VariableName=mc_hoist_integral2  SaveFormat=Timeseries  SampleTime=-1
      settings: Decimation=10
  RegistroPersistente_574 : ToWorkspace  VariableName=mc_hoist_P  SaveFormat=Timeseries  SampleTime=-1
      settings: Decimation=10
  RegistroPersistente_575 : ToWorkspace  VariableName=mc_hoist_D  SaveFormat=Timeseries  SampleTime=-1
      settings: Decimation=10
  RegistroPersistente_576 : ToWorkspace  VariableName=mc_hoist_I  SaveFormat=Timeseries  SampleTime=-1
      settings: Decimation=10
  RegistroPersistente_577 : ToWorkspace  VariableName=mc_hoist_FF  SaveFormat=Timeseries  SampleTime=-1
      settings: Decimation=10
  wires:
  Diagnosticos izaje selector/6 -> Monitor mc_hoist_D/1, RegistroPersistente_575/1  "<mc_hoist_D>"
  Diagnosticos carro selector/27 -> Monitor diag_aref_input/1, RegistroPersistente_564/1  "<diag_aref_input>"
  In1/1 -> Diagnosticos carro selector/1
  Diagnosticos carro selector/22 -> Monitor diag_sw_gain/1, RegistroPersistente_559/1  "<diag_sw_gain>"
  Diagnosticos izaje selector/5 -> Monitor mc_hoist_P/1, RegistroPersistente_574/1  "<mc_hoist_P>"
  Diagnosticos carro selector/3 -> Monitor diag_vcmd_applied/1, RegistroPersistente_540/1  "<diag_vcmd_applied>"
  Diagnosticos carro selector/18 -> Monitor sw_feedback_comun/1, RegistroPersistente_555/1  "<sw_feedback_comun>"
  Diagnosticos carro selector/4 -> Monitor diag_vobs/1, RegistroPersistente_541/1  "<diag_vobs>"
  Diagnosticos carro selector/15 -> Monitor aw_correccion_integrador/1, RegistroPersistente_552/1  "<aw_correccion_integrador>"
  In2/1 -> Diagnosticos izaje selector/1
  Diagnosticos carro selector/21 -> Monitor diag_sw_unsat/1, RegistroPersistente_558/1  "<diag_sw_unsat>"
  Diagnosticos carro selector/9 -> Monitor diag_acmd_applied/1, RegistroPersistente_546/1  "<diag_acmd_applied>"
  Diagnosticos carro selector/12 -> Monitor aw_delta_a_limite_memoria/1, RegistroPersistente_549/1  "<aw_delta_a_limite_memoria>"
  Diagnosticos carro selector/7 -> Monitor diag_i/1, RegistroPersistente_544/1  "<diag_i>"
  Diagnosticos carro selector/8 -> Monitor diag_acmd/1, RegistroPersistente_545/1  "<diag_acmd>"
  Diagnosticos carro selector/6 -> Monitor diag_p/1, RegistroPersistente_543/1  "<diag_p>"
  Diagnosticos carro selector/20 -> Monitor sw_habilitacion_comun/1, RegistroPersistente_557/1  "<sw_habilitacion_comun>"
  Diagnosticos carro selector/19 -> Monitor sw_anticipacion_comun/1, RegistroPersistente_556/1  "<sw_anticipacion_comun>"
  Diagnosticos carro selector/26 -> Monitor diag_vref_input/1, RegistroPersistente_563/1  "<diag_vref_input>"
  Diagnosticos carro selector/11 -> Monitor aw_delta_a_limite/1, RegistroPersistente_548/1  "<aw_delta_a_limite>"
  Diagnosticos carro selector/32 -> Monitor diag_brake_supervisor/1, RegistroPersistente_569/1  "<diag_brake_supervisor>"
  Diagnosticos carro selector/13 -> Monitor aw_delta_a_torque/1, RegistroPersistente_550/1  "<aw_delta_a_torque>"
  Diagnosticos carro selector/2 -> Monitor diag_vcmd/1, RegistroPersistente_539/1  "<diag_vcmd>"
  Diagnosticos carro selector/17 -> Monitor antisway_correccion_aplicada/1, RegistroPersistente_554/1  "<antisway_correccion_aplicada>"
  Diagnosticos izaje selector/1 -> Monitor torque_izaje_consigna_controlador/1, RegistroPersistente_570/1  "<torque_izaje_consigna_controlador>"
  Diagnosticos carro selector/10 -> Monitor diag_ev/1, RegistroPersistente_547/1  "<diag_ev>"
  Diagnosticos carro selector/1 -> Monitor diag_torque_unsat/1, RegistroPersistente_538/1  "<diag_torque_unsat>"
  Diagnosticos carro selector/5 -> Monitor diag_integral/1, RegistroPersistente_542/1  "<diag_integral>"
  Diagnosticos carro selector/16 -> Monitor mc_integrator_input/1, RegistroPersistente_553/1  "<mc_integrator_input>"
  Diagnosticos izaje selector/4 -> Monitor mc_hoist_integral2/1, RegistroPersistente_573/1  "<mc_hoist_integral2>"
  Diagnosticos izaje selector/2 -> Monitor mc_hoist_velocity_error/1, RegistroPersistente_571/1  "<mc_hoist_velocity_error>"
  Diagnosticos izaje selector/3 -> Monitor mc_hoist_integral1/1, RegistroPersistente_572/1  "<mc_hoist_integral1>"
  Diagnosticos carro selector/14 -> Monitor aw_delta_a_total/1, RegistroPersistente_551/1  "<aw_delta_a_total>"
  Diagnosticos carro selector/28 -> Monitor diag_xencoder/1, RegistroPersistente_565/1  "<diag_xencoder>"
  Diagnosticos carro selector/24 -> Monitor diag_aff/1, RegistroPersistente_561/1  "<diag_aff>"
  Diagnosticos carro selector/23 -> Monitor angulo_referencia/1, RegistroPersistente_560/1  "<angulo_referencia>"
  Diagnosticos carro selector/30 -> Monitor diag_theta_medida/1, RegistroPersistente_567/1  "<diag_theta_medida>"
  Diagnosticos carro selector/31 -> Monitor diag_theta_eff/1, RegistroPersistente_568/1  "<diag_theta_eff>"
  Diagnosticos carro selector/29 -> Monitor diag_omega_observer/1, RegistroPersistente_566/1  "<diag_omega_observer>"
  Diagnosticos carro selector/25 -> Monitor diag_xref_input/1, RegistroPersistente_562/1  "<diag_xref_input>"
  Diagnosticos izaje selector/8 -> Monitor mc_hoist_FF/1, RegistroPersistente_577/1  "<mc_hoist_FF>"
  Diagnosticos izaje selector/7 -> Monitor mc_hoist_I/1, RegistroPersistente_576/1  "<mc_hoist_I>"

== system Grua_MC_R2_FFLimitado_06102026/Planta/Calculo longitud l ==
  x_l : Inport
  y_l : Inport  Port=2
  v_lx : Inport  Port=3
  v_ly : Inport  Port=4
  x_t : Inport  Port=5
  v_t : Inport  Port=6
  Constant : Constant  Value=Y_t0
  Divide : Product  Inputs=*/
  Product : Product
  Product1 : Product
  Sqrt : Sqrt
  Square : Math  Operator=square
  Square1 : Math  Operator=square
  Sum : Sum  Inputs=|+-
  Sum1 : Sum  Inputs=|+-
  Sum2 : Sum
  Sum3 : Sum  Inputs=|+-
  Sum4 : Sum  Inputs=+-
  l : Outport
  dl : Outport  Port=2
  wires:
  Sqrt/1 -> Divide/2, l/1  "l"
  x_l/1 -> Sum/1
  x_t/1 -> Sum/2
  Sum/1 -> Product/1, Square/1
  Constant/1 -> Sum1/1
  y_l/1 -> Sum1/2
  Sum1/1 -> Product1/1, Square1/1
  Square1/1 -> Sum2/2
  Square/1 -> Sum2/1
  Sum2/1 -> Sqrt/1
  v_lx/1 -> Sum3/1
  v_t/1 -> Sum3/2
  Sum3/1 -> Product/2
  v_ly/1 -> Product1/2
  Product1/1 -> Sum4/2
  Product/1 -> Sum4/1
  Sum4/1 -> Divide/1
  Divide/1 -> dl/1  "dl"

== system Grua_MC_R2_FFLimitado_06102026/Planta/Subsistema carga ==
  x_t : Inport
  F_w : Inport  Port=2
  M_c : Inport  Port=3
  y_c0(x_l,t) : Inport  Port=4
  TLK : Inport  Port=5
  Calculo Angulo De Balanceo : Subsystem
  Calculo Fuerza De Contacto : Subsystem
  Calculo Longitud Inferior : Subsystem
  Calculo Masa Total de Carga : Subsystem
  Derivative : Derivative
  Dinamica Movimiento Carga : Subsystem
  RegistroPersistente_730 : ToWorkspace  VariableName=masa_fisica_suspendida  SaveFormat=Timeseries  SampleTime=-1
      settings: Decimation=10
  RegistroPersistente_738 : ToWorkspace  VariableName=y_carga_fisica  SaveFormat=Timeseries  SampleTime=-1
      settings: Decimation=10
  RegistroPersistente_740 : ToWorkspace  VariableName=v_izaje_fisica  SaveFormat=Timeseries  SampleTime=-1
      settings: Decimation=10
  x_l : Outport
  y_l : Outport  Port=2
  v_lx : Outport  Port=3
  v_ly : Outport  Port=4
  theta_l : Outport  Port=5
  omega_l : Outport  Port=6
  F_cy : Outport  Port=7
  wires:
  Calculo Fuerza De Contacto/2(F_cy) -> F_cy/1, Dinamica Movimiento Carga/3(F_cy)
  Dinamica Movimiento Carga/4(v_ly) -> v_ly/1, Calculo Fuerza De Contacto/3(v_ly), RegistroPersistente_740/1
  x_t/1 -> Calculo Angulo De Balanceo/3(x_t)
  Dinamica Movimiento Carga/2(y_l) -> y_l/1, Calculo Angulo De Balanceo/2(y_l), Calculo Fuerza De Contacto/1(y_l), RegistroPersistente_738/1
  Calculo Angulo De Balanceo/1(theta_l) -> Dinamica Movimiento Carga/5(theta_l), Derivative/1, theta_l/1
  y_c0(x_l,t)/1 -> Calculo Fuerza De Contacto/5(y_c0(x_l,t))
  Calculo Fuerza De Contacto/1(F_cx) -> Dinamica Movimiento Carga/2(F_cx)
  Dinamica Movimiento Carga/1(x_l) -> x_l/1, Calculo Angulo De Balanceo/1(x_l)
  Dinamica Movimiento Carga/3(v_lx) -> v_lx/1, Calculo Fuerza De Contacto/2(v_lx)
  Calculo Longitud Inferior/1(h_c) -> Calculo Fuerza De Contacto/4(h_c)
  F_w/1 -> Dinamica Movimiento Carga/4(F_hw)
  M_c/1 -> Calculo Masa Total de Carga/2(M_c)
  TLK/1 -> Calculo Longitud Inferior/1(TLK), Calculo Masa Total de Carga/1(TLK)
  Derivative/1 -> omega_l/1
  Calculo Masa Total de Carga/1(m_l) -> Dinamica Movimiento Carga/1(m_l), RegistroPersistente_730/1

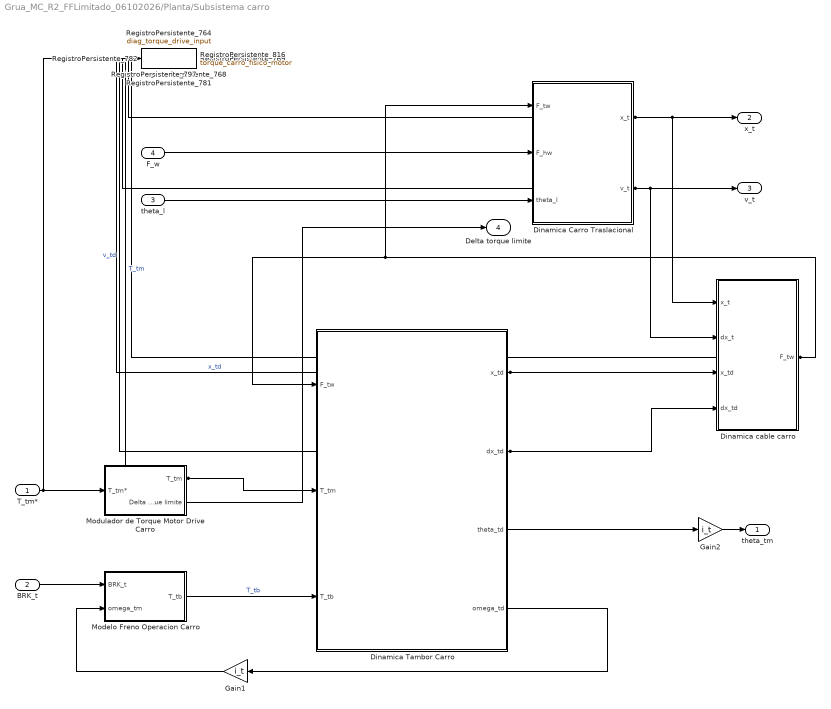
== system Grua_MC_R2_FFLimitado_06102026/Planta/Subsistema carro ==
  T_tm* : Inport
  BRK_t : Inport  Port=2
  theta_l : Inport  Port=3
  F_w : Inport  Port=4
  Dinamica Carro Traslacional : Subsystem
  Dinamica Tambor Carro : Subsystem
  Dinamica cable carro : Subsystem
  Gain1 : Gain  Gain=i_t
  Gain2 : Gain  Gain=i_t
  Modelo Freno Operacion Carro : Subsystem
  Modulador de Torque Motor Drive Carro : Subsystem
  RegistroPersistente_764 : ToWorkspace  VariableName=diag_torque_drive_input  SaveFormat=Timeseries  SampleTime=-1
      settings: Decimation=10
  RegistroPersistente_768 : ToWorkspace  VariableName=x_carro_fisica  SaveFormat=Timeseries  SampleTime=-1
      settings: Decimation=10
  RegistroPersistente_769 : ToWorkspace  VariableName=v_carro_fisica  SaveFormat=Timeseries  SampleTime=-1
      settings: Decimation=10
  RegistroPersistente_781 : ToWorkspace  VariableName=x_td  SaveFormat=Timeseries  SampleTime=-1
      settings: Decimation=10
  RegistroPersistente_782 : ToWorkspace  VariableName=v_td  SaveFormat=Timeseries  SampleTime=-1
      settings: Decimation=10
  RegistroPersistente_797 : ToWorkspace  VariableName=diag_traction  SaveFormat=Timeseries  SampleTime=-1
      settings: Decimation=10
  RegistroPersistente_816 : ToWorkspace  VariableName=torque_carro_fisico_motor  SaveFormat=Timeseries  SampleTime=-1
      settings: Decimation=10
  theta_tm : Outport
  x_t : Outport  Port=2
  v_t : Outport  Port=3
  Delta torque limite : Outport  Port=4
  wires:
  Dinamica cable carro/1(F_tw) -> Dinamica Carro Traslacional/1(F_tw), Dinamica Tambor Carro/1(F_tw), RegistroPersistente_797/1
  Gain1/1 -> Modelo Freno Operacion Carro/2(omega_tm)
  F_w/1 -> Dinamica Carro Traslacional/2(F_hw)
  Dinamica Carro Traslacional/1(x_t) -> x_t/1, Dinamica cable carro/1(x_t), RegistroPersistente_768/1
  Modulador de Torque Motor Drive Carro/1(T_tm) -> Dinamica Tambor Carro/2(T_tm), RegistroPersistente_816/1  "T_tm"
  Dinamica Tambor Carro/4(omega_td) -> Gain1/1
  Dinamica Carro Traslacional/2(v_t) -> v_t/1, Dinamica cable carro/2(dx_t), RegistroPersistente_769/1
  Dinamica Tambor Carro/2(dx_td) -> Dinamica cable carro/4(dx_td), RegistroPersistente_782/1  "v_td"
  Dinamica Tambor Carro/1(x_td) -> Dinamica cable carro/3(x_td), RegistroPersistente_781/1  "x_td"
  Modelo Freno Operacion Carro/1(T_tb) -> Dinamica Tambor Carro/3(T_tb)  "T_tb"
  BRK_t/1 -> Modelo Freno Operacion Carro/1(BRK_t)
  Dinamica Tambor Carro/3(theta_td) -> Gain2/1
  T_tm*/1 -> Modulador de Torque Motor Drive Carro/1(T_tm*), RegistroPersistente_764/1
  theta_l/1 -> Dinamica Carro Traslacional/3(theta_l)
  Gain2/1 -> theta_tm/1
  Modulador de Torque Motor Drive Carro/2(Delta torque limite) -> Delta torque limite/1

== system Grua_MC_R2_FFLimitado_06102026/Planta/Subsistema izaje ==
  F_hw : Inport
  BRK_hE : Inport  Port=2
  T_hm* : Inport  Port=3
  BRK_h : Inport  Port=4
  l : Inport  Port=5
  dl : Inport  Port=6
  Calculo longitud l_h : Subsystem
  Dinamica Tambor Izaje : Subsystem
  Dinamica cable Izaje : Subsystem
  Gain : Gain  Gain=i_h
  Gain1 : Gain  Gain=i_h
  Modelo Freno Emergencia de Izaje(Eje lento) : Subsystem
  Modelo Freno Operacion de Izaje(Eje Rapido) : Subsystem
  Modulador de Torque Motor Drive Izaje : Subsystem
  RegistroPersistente_834 : ToWorkspace  VariableName=l_h  SaveFormat=Timeseries  SampleTime=-1
      settings: Decimation=10
  RegistroPersistente_892 : ToWorkspace  VariableName=torque_izaje_fisico_motor  SaveFormat=Timeseries  SampleTime=-1
      settings: Decimation=10
  theta_hd : Outport
  theta_hm : Outport  Port=2
  F_w : Outport  Port=3
  omega_hd : Outport  Port=4
  wires:
  Calculo longitud l_h/1(l_h) -> Dinamica cable Izaje/2(l_h), RegistroPersistente_834/1  "l_h"
  Calculo longitud l_h/2(dl_h) -> Dinamica cable Izaje/4(dl_h)
  F_hw/1 -> Dinamica Tambor Izaje/3(F_hw)
  Modelo Freno Emergencia de Izaje(Eje lento)/1(T_hEb) -> Dinamica Tambor Izaje/1(T_hEb)
  Dinamica Tambor Izaje/1(theta_hd) -> Gain1/1, theta_hd/1
  BRK_h/1 -> Modelo Freno Operacion de Izaje(Eje Rapido)/1(BRK_h)
  Modelo Freno Operacion de Izaje(Eje Rapido)/1(T_hb) -> Dinamica Tambor Izaje/4(T_hb)
  Gain/1 -> Modulador de Torque Motor Drive Izaje/2(omega_hm), Modelo Freno Operacion de Izaje(Eje Rapido)/2(omega_hm)
  BRK_hE/1 -> Modelo Freno Emergencia de Izaje(Eje lento)/2(BRK_hE)
  T_hm*/1 -> Modulador de Torque Motor Drive Izaje/1(T_hm*)
  l/1 -> Dinamica cable Izaje/1(l)
  Dinamica cable Izaje/1(F_hw) -> F_w/1  "F_w"
  dl/1 -> Dinamica cable Izaje/3(dl)
  Modulador de Torque Motor Drive Izaje/1(T_hm) -> Dinamica Tambor Izaje/2(T_hm), RegistroPersistente_892/1
  Gain1/1 -> theta_hm/1
  Dinamica Tambor Izaje/2(omega_hd) -> Gain/1, Modelo Freno Emergencia de Izaje(Eje lento)/1(omega_hd), Calculo longitud l_h/1(omega_hd), omega_hd/1

== system Grua_MC_R2_FFLimitado_06102026/SENSORES/Finales de carrera operacion carro ==
  x_t : Inport
  Constant : Constant  Value=x_tmax
  Constant1 : Constant  Value=x_tmin
  Constant2 : Constant  Value=x_tmax+0.50
  Constant3 : Constant  Value=x_tmin-0.50
  Relational Operator{1..4} (4 alike) : RelationalOperator  OutDataTypeStr=boolean  RndMeth=Simplest  InputSameDT=off
  x_tLSmax : Outport
  x_tLSmin : Outport  Port=2
  x_tLSEmax : Outport  Port=3
  x_tLSEmin : Outport  Port=4
  wires:
  Relational Operator4/1 -> x_tLSmax/1
  Constant/1 -> Relational Operator4/2
  Constant1/1 -> Relational Operator1/1
  x_t/1 -> Relational Operator3/2, Relational Operator2/1, Relational Operator1/2, Relational Operator4/1
  Relational Operator1/1 -> x_tLSmin/1
  Relational Operator3/1 -> x_tLSEmin/1
  Relational Operator2/1 -> x_tLSEmax/1
  Constant2/1 -> Relational Operator2/2
  Constant3/1 -> Relational Operator3/1

== system Grua_MC_R2_FFLimitado_06102026/SENSORES/Sensor de Sobrevelocidad>115% ==
  v_h : Inport
  TLK : Inport  Port=2
  Abs : Abs  SaturateOnIntegerOverflow=off
  Constant : Constant  Value=v_hmaxLoaded
  Constant1 : Constant  Value=v_hmaxUnloaded
  Gain : Gain  Gain=1.15
  Relational Operator : RelationalOperator  OutDataTypeStr=boolean  RndMeth=Simplest  InputSameDT=off
  Switch : Switch  Criteria=u2 > Threshold  SaturateOnIntegerOverflow=off  InputSameDT=off
  Sobrevelocidad : Outport
  wires:
  Switch/1 -> Gain/1  "v_hlim"
  Constant/1 -> Switch/1
  TLK/1 -> Switch/2
  Constant1/1 -> Switch/3
  v_h/1 -> Abs/1
  Relational Operator/1 -> Sobrevelocidad/1
  Gain/1 -> Relational Operator/2
  Abs/1 -> Relational Operator/1

== system Grua_MC_R2_FFLimitado_06102026/SENSORES/Subsystem1 ==
  theta_l : Inport
  omega_l : Inport  Port=2
  sensor angulo vertical : Gain
  sensor de velocidad angular : Gain
  theta_l_sensor : Outport
  omega_l_sensor : Outport  Port=2
  wires:
  sensor angulo vertical/1 -> theta_l_sensor/1
  sensor de velocidad angular/1 -> omega_l_sensor/1
  omega_l/1 -> sensor de velocidad angular/1
  theta_l/1 -> sensor angulo vertical/1

== system Grua_MC_R2_FFLimitado_06102026/Planta/Subsistema carga/Calculo Angulo De Balanceo ==
  x_l : Inport
  y_l : Inport  Port=2
  x_t : Inport  Port=3
  Atan : Trigonometry  Operator=atan2
  Constant : Constant  Value=Y_t0
  RegistroPersistente_702 : ToWorkspace  VariableName=x_l  SaveFormat=Timeseries  SampleTime=-1
      settings: Decimation=10
  RegistroPersistente_703 : ToWorkspace  VariableName=y_l  SaveFormat=Timeseries  SampleTime=-1
      settings: Decimation=10
  RegistroPersistente_704 : ToWorkspace  VariableName=x_t  SaveFormat=Timeseries  SampleTime=-1
      settings: Decimation=10
  Sum : Sum  Inputs=|+-
  Sum1 : Sum  Inputs=|+-
  theta_l : Outport
  wires:
  x_l/1 -> Sum/1, RegistroPersistente_702/1  "x_l"
  x_t/1 -> Sum/2, RegistroPersistente_704/1  "x_t"
  Constant/1 -> Sum1/1
  y_l/1 -> Sum1/2, RegistroPersistente_703/1  "y_l"
  Sum/1 -> Atan/1
  Sum1/1 -> Atan/2
  Atan/1 -> theta_l/1

== system Grua_MC_R2_FFLimitado_06102026/Planta/Subsistema carga/Calculo Fuerza De Contacto ==
  y_l : Inport
  v_lx : Inport  Port=2
  v_ly : Inport  Port=3
  h_c : Inport  Port=4
  y_c0(x_l,t) : Inport  Port=5
  Constant1 : Constant  Value=0
  Gain : Gain  Gain=-b_cx
  Gain1 : Gain  Gain=K_cy
  Gain2 : Gain  Gain=-b_cy
  Limite fuerza contacto : Saturate  UpperLimit=2e6  LowerLimit=0
  RegistroPersistente_721 : ToWorkspace  VariableName=sumFcx  SaveFormat=Timeseries  SampleTime=-1
      settings: Decimation=10
  RegistroPersistente_723 : ToWorkspace  VariableName=registro_723  SaveFormat=Timeseries  SampleTime=-1
      settings: Decimation=10
  Sum : Sum  Inputs=++-
  Sum1 : Sum  Inputs=|++
  Switch : Switch  SaturateOnIntegerOverflow=off  InputSameDT=off
  Switch1 : Switch  SaturateOnIntegerOverflow=off  InputSameDT=off
  F_cx : Outport
  F_cy : Outport  Port=2
  wires:
  Switch/1 -> F_cx/1, RegistroPersistente_723/1
  Constant1/1 -> Switch1/3, Switch/3
  Gain/1 -> Switch/1
  h_c/1 -> Sum/2
  y_c0(x_l,t)/1 -> Sum/1
  y_l/1 -> Sum/3
  Sum/1 -> Gain1/1, Switch1/2, Switch/2, RegistroPersistente_721/1  "sumFcx"
  v_lx/1 -> Gain/1
  Gain1/1 -> Sum1/1
  Gain2/1 -> Sum1/2
  v_ly/1 -> Gain2/1
  Sum1/1 -> Switch1/1
  Switch1/1 -> Limite fuerza contacto/1
  Limite fuerza contacto/1 -> F_cy/1

== system Grua_MC_R2_FFLimitado_06102026/Planta/Subsistema carga/Calculo Longitud Inferior ==
  TLK : Inport
  Constant : Constant  Value=H_c
  Constant1 : Constant  Value=0
  Switch : Switch  Criteria=u2 > Threshold  SaturateOnIntegerOverflow=off  InputSameDT=off
  h_c : Outport
  wires:
  TLK/1 -> Switch/2
  Switch/1 -> h_c/1
  Constant1/1 -> Switch/3
  Constant/1 -> Switch/1

== system Grua_MC_R2_FFLimitado_06102026/Planta/Subsistema carga/Calculo Masa Total de Carga ==
  TLK : Inport
  M_c : Inport  Port=2
  Constant : Constant  Value=M_s
  RegistroPersistente_735 : ToWorkspace  VariableName=masa_total_fisica  SaveFormat=Timeseries  SampleTime=-1
      settings: Decimation=10
  Sum : Sum  Inputs=|++
  Switch : Switch  Criteria=u2 > Threshold  SaturateOnIntegerOverflow=off  InputSameDT=off
  m_l : Outport
  wires:
  TLK/1 -> Switch/2
  M_c/1 -> Sum/2
  Switch/1 -> m_l/1, RegistroPersistente_735/1
  Constant/1 -> Sum/1, Switch/3
  Sum/1 -> Switch/1
